simulink model "segway"  (R2020a)
settings: Solver=VariableStepAuto  StartTime=0.0  StopTime=0.2  RelTol=1e-5
values from neighbouring files (symbols this model uses):
  D = [0 0;     0 0;     0 0;     0 0]    [data.m]    (also in segway.mat = 0.15)
  g = 9.81    [segway.mat]
  J_o = 2.023e-05    [segway.mat]
  J_p = 0.0016    [segway.mat]
  J_phi = 0.00143    [segway.mat]
  k_e = 0.005    [segway.mat]
  k_m = 0.0019    [segway.mat]
  L = 0.07    [segway.mat]
  M = 0.035    [segway.mat]
  m = 0.81    [segway.mat]
  R = [0.03 0;     0 0.02]    [data.m]    (also in segway.mat = 0.034)
  R_e = 0.36    [segway.mat]
settings Model: Creator=dell  LastModifiedBy=dell
settings SolverCC: AlgebraicLoopSolver=LineSearch

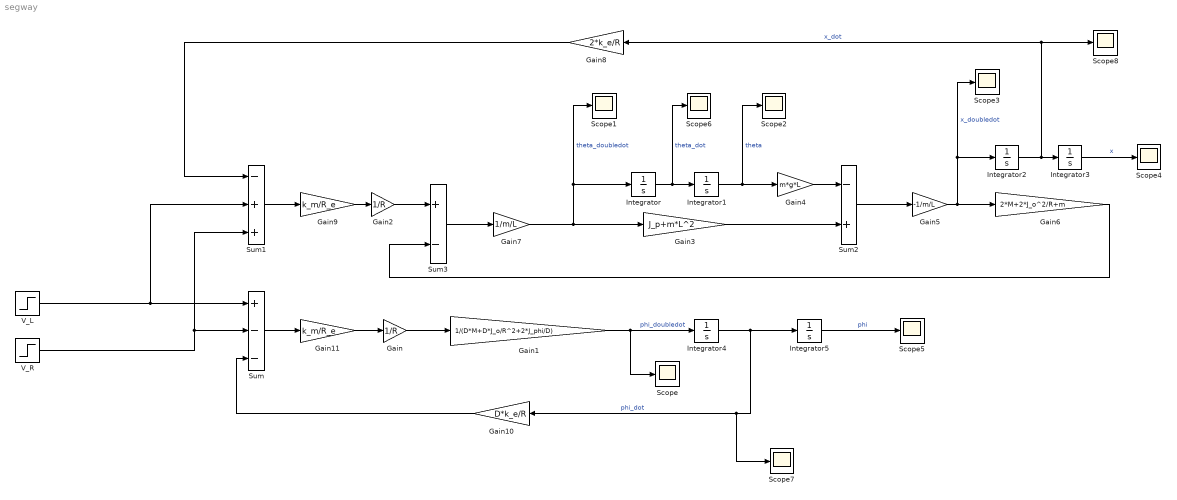
== system segway ==
  Gain : Gain  Gain=1/R
  Gain1 : Gain  Gain=1/(D*M+D*J_o/R^2+2*J_phi/D)
  Gain10 : Gain  Gain=D*k_e/R
  Gain11 : Gain  Gain=k_m/R_e
  Gain2 : Gain  Gain=1/R
  Gain3 : Gain  Gain=J_p+m*L^2
  Gain4 : Gain  Gain=m*g*L
  Gain5 : Gain  Gain=-1/m/L
  Gain6 : Gain  Gain=2*M+2*J_o^2/R+m
  Gain7 : Gain  Gain=1/m/L
  Gain8 : Gain  Gain=2*k_e/R
  Gain9 : Gain  Gain=k_m/R_e
  Integrator{,2..4} (4 alike) : Integrator
  Integrator1 : Integrator  LimitOutput=on  UpperSaturationLimit=pi/2  LowerSaturationLimit=-pi/2
  Integrator5 : Integrator  UpperSaturationLimit=2*pi  LowerSaturationLimit=0
  Scope{,1..8} (9 alike) : Scope
  Sum : Sum  Inputs=+--
  Sum1 : Sum  Inputs=-++
  Sum2 : Sum  Inputs=-+
  Sum3 : Sum  Inputs=+-
  V_L : Step  Time=0  After=6  SampleTime=0
  V_R : Step  Time=0  After=3  SampleTime=0
  wires:
  V_L/1 -> Sum1/2, Sum/1
  V_R/1 -> Sum1/3, Sum/2
  Gain/1 -> Gain1/1
  Sum1/1 -> Gain9/1
  Sum2/1 -> Gain5/1
  Gain5/1 -> Gain6/1, Integrator2/1, Scope3/1  "x_doubledot"
  Gain2/1 -> Sum3/1
  Gain6/1 -> Sum3/2
  Sum3/1 -> Gain7/1
  Gain3/1 -> Sum2/2
  Gain4/1 -> Sum2/1
  Gain7/1 -> Scope1/1, Integrator/1, Gain3/1  "theta_doubledot"
  Integrator1/1 -> Scope2/1, Gain4/1  "theta"
  Integrator3/1 -> Scope4/1  "x"
  Gain1/1 -> Integrator4/1, Scope/1  "phi_doubledot"
  Gain8/1 -> Sum1/1
  Gain9/1 -> Gain2/1
  Gain10/1 -> Sum/3
  Integrator5/1 -> Scope5/1  "phi"
  Gain11/1 -> Gain/1
  Sum/1 -> Gain11/1
  Integrator/1 -> Scope6/1, Integrator1/1  "theta_dot"
  Integrator4/1 -> Scope7/1, Gain10/1, Integrator5/1  "phi_dot"
  Integrator2/1 -> Gain8/1, Scope8/1, Integrator3/1  "x_dot"
